simulink model "F_A"  (R2013a)
settings: Solver=ode45  StartTime=0.0  StopTime=0.2  RelTol=1e-3
settings Model: Creator=MEHEDI HASSAN  LastModifiedBy=MEHEDI HASSAN
settings OptimizationCC: InlineParams=on
settings DebuggingCC: SolverPrmCheckMsg=none  ModelReferenceExtraNoncontSigs=none

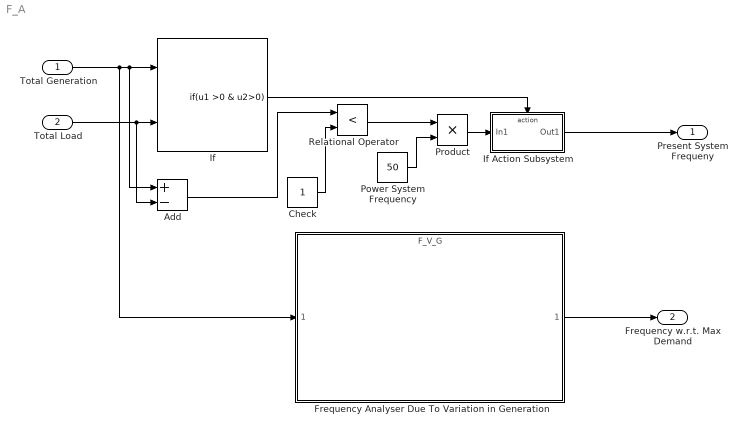
== system F_A ==
  Total Generation : Inport
  Total Load : Inport  Port=2
  Add : Sum  Inputs=+-
  Check : Constant
  Frequency Analyser Due To Variation in Generation : ModelReference  ModelNameDialog=F_V_G.slx  SimulationMode=Normal  ModelReferenceVersion=1.5  CopyOfModelName=F_V_G.slx  DefaultDataLogging=on
  If : If  NumInputs=2  IfExpression=u1 >0 & u2>0  ShowElse=off
  If Action Subsystem : Subsystem  TreatAsAtomicUnit=on
  Power System Frequency : Constant  Value=50
  Product : Product
  Relational Operator : RelationalOperator  Operator=<  OutDataTypeStr=boolean
  Present System Frequeny : Outport
  Frequency w.r.t. Max Demand : Outport  Port=2
  wires:
  If/1 -> If Action Subsystem/Action
  Total Generation/1 -> Frequency Analyser Due To Variation in Generation/1, Add/1, If/1
  Total Load/1 -> Add/2, If/2
  If Action Subsystem/1(Out1) -> Present System Frequeny/1
  Frequency Analyser Due To Variation in Generation/1 -> Frequency w.r.t. Max Demand/1
  Check/1 -> Relational Operator/2
  Relational Operator/1 -> Product/1
  Power System Frequency/1 -> Product/2
  Product/1 -> If Action Subsystem/1(In1)
  Add/1 -> Relational Operator/1

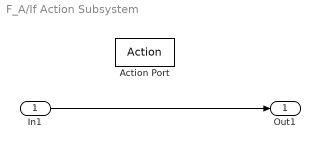
== system F_A/If Action Subsystem ==
  In1 : Inport
  Action Port : ActionPort  ActionType=then
  Out1 : Outport
  wires:
  In1/1 -> Out1/1
